simulink model "PIControllerModel"  (R2024b)
settings: Solver=VariableStepAuto  StartTime=0.0  StopTime=10  RelTol=1e-3
values from neighbouring files (symbols this model uses):
  c = 160e-6    (= 0.00016)    [ParamTestSimulationDroop.m]    (also in ParamTestSimulatitestFirstandPI.m)
  Kp_currentLoop = X*r    (= 0.5)    [ParamTestSimulationDroop.m]    (also in ParamTestSimulatitestFirstandPI.m)
  Kp_voltageLoop = Xvoltage/Rc    (= 0.005)    [ParamTestSimulationDroop.m]    (also in ParamTestSimulatitestFirstandPI.m)
  l = 300e-6    (= 0.0003)    [ParamTestSimulationDroop.m]    (also in ParamTestSimulatitestFirstandPI.m)
  r = 0.1    [ParamTestSimulationDroop.m]    (also in ParamTestSimulatitestFirstandPI.m)
  Rc = 1e3    (= 1000)    [ParamTestSimulationDroop.m]    (also in ParamTestSimulatitestFirstandPI.m)
  T32 = sqrt(2/3)*[1 0;-1/2 sqrt(3)/2;-1/2 -sqrt(3)/2]    [ParamTestSimulationDroop.m]    (also in ParamTestSimulatitestFirstandPI.m)
  towI_currentLoop = tow_currnet    (= 0.003)    [ParamTestSimulationDroop.m]    (also in ParamTestSimulatitestFirstandPI.m)
  towI_voltageLoop = tow_voltage    (= 0.16)    [ParamTestSimulationDroop.m]    (also in ParamTestSimulatitestFirstandPI.m)
libraries: spsThreePhaseSeriesRLCBranchLib x7, spsControlledVoltageSourceLib x3, spsThreePhaseVIMeasurementLib x2, spsGroundLib x1, sps_lib x1
settings Model: Creator=manip  LastModifiedBy=rashi
settings SolverCC: AlgebraicLoopSolver=TrustRegion
settings DebuggingCC: UnconnectedInputMsg=warning  UnconnectedOutputMsg=warning  UnconnectedLineMsg=warning
settings ModelReferenceCC: EnableRefExpFcnMdlSchedulingChecks=on
settings RTWCC: GPUComputeCapability=3.5

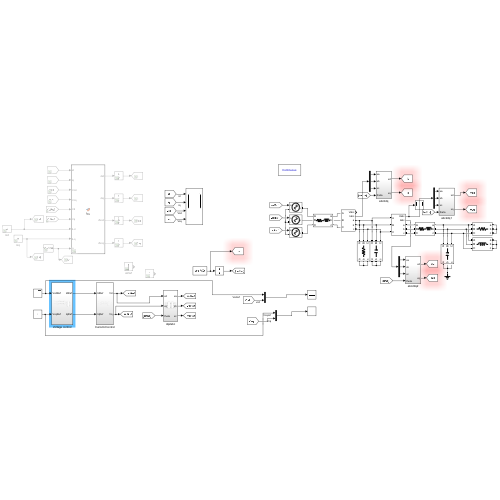
[thumbnail: Simulink's stored preview of the top-level diagram]
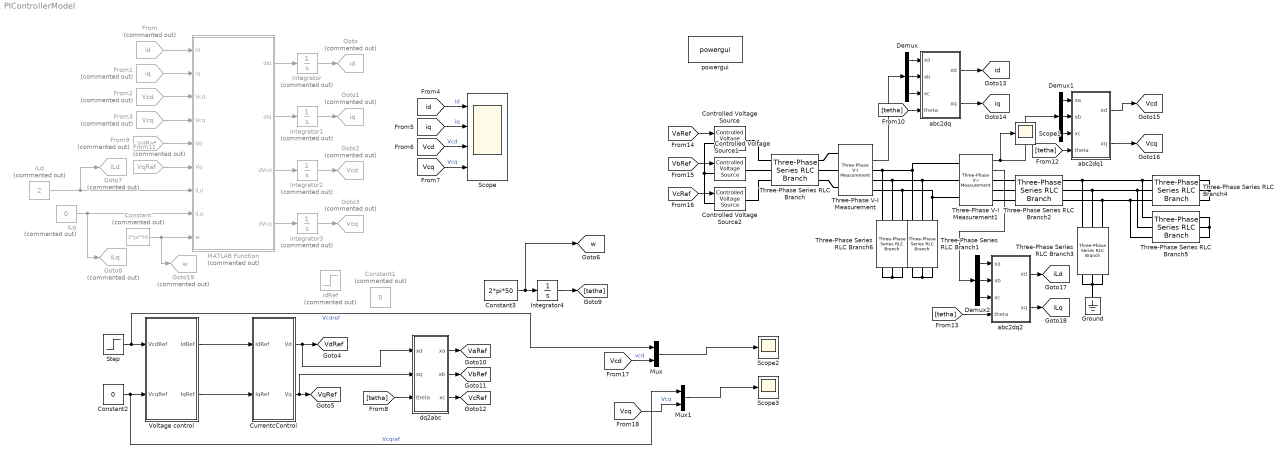
== system PIControllerModel ==
  Constant : Constant  Commented=on  Value=2*pi*50
  Constant1 : Constant  Commented=on  Value=0
  Constant2 : Constant  Value=0
  Constant3 : Constant  Value=2*pi*50
  Controlled Voltage Source : spsControlledVoltageSourceLib/Controlled Voltage Source  Initialize=on  Source_Type=AC  Amplitude=0  Phase=0  Frequency=0  Measurements=None
  Controlled Voltage Source1 : spsControlledVoltageSourceLib/Controlled Voltage Source  Initialize=on  Source_Type=AC  Amplitude=0  Phase=0  Frequency=0  Measurements=None
  Controlled Voltage Source2 : spsControlledVoltageSourceLib/Controlled Voltage Source  Initialize=on  Source_Type=AC  Amplitude=0  Phase=0  Frequency=0  Measurements=None
  CurrentcControl : Subsystem
  Demux : Demux  Outputs=3
  Demux1 : Demux  Outputs=3
  Demux2 : Demux  Outputs=3
  From : From  Commented=on  GotoTag=id  TagVisibility=global
  From1 : From  Commented=on  GotoTag=iq  TagVisibility=global
  From11 : From  Commented=on  GotoTag=VqRef  TagVisibility=global
  From2 : From  Commented=on  GotoTag=Vcd  TagVisibility=global
  From3 : From  Commented=on  GotoTag=Vcq  TagVisibility=global
  From9 : From  Commented=on  GotoTag=VdRef  TagVisibility=global
  Goto : Goto  Commented=on  GotoTag=id  TagVisibility=global
  Goto1 : Goto  Commented=on  GotoTag=iq  TagVisibility=global
  Goto19 : Goto  Commented=on  GotoTag=w  TagVisibility=global
  Goto2 : Goto  Commented=on  GotoTag=Vcd  TagVisibility=global
  Goto3 : Goto  Commented=on  GotoTag=Vcq  TagVisibility=global
  Goto7 : Goto  Commented=on  GotoTag=iLd  TagVisibility=global
  Goto8 : Goto  Commented=on  GotoTag=iLq  TagVisibility=global
  Ground : spsGroundLib/Ground  LConnTagsString=a
  Integrator{,1..3} (4 alike) : Integrator  Commented=on
  Integrator4 : Integrator
  MATLAB Function : MATLAB Function  Commented=on  TreatAsAtomicUnit=on
  Mux : Mux  Inputs=2
  Mux1 : Mux  Inputs=2
  Scope : Scope  NumInputPorts=4
  Scope1 : Scope
  Scope2 : Scope
  Scope3 : Scope
  Step : Step  Time=3  Before=50  After=110  SampleTime=0
  Three-Phase Series RLC Branch : spsThreePhaseSeriesRLCBranchLib/Three-Phase Series RLC Branch  LConnTagsString=A|B|C  RConnTagsString=A|B|C  BranchType=RL  Resistance=r  Inductance=l  Capacitance=1e-6  Measurements=None
  Three-Phase Series RLC Branch1 : spsThreePhaseSeriesRLCBranchLib/Three-Phase Series RLC Branch  LConnTagsString=A|B|C  RConnTagsString=A|B|C  BranchType=C  Resistance=r  Inductance=l  Capacitance=c  Measurements=None
  Three-Phase Series RLC Branch2 : spsThreePhaseSeriesRLCBranchLib/Three-Phase Series RLC Branch  LConnTagsString=A|B|C  RConnTagsString=A|B|C  BranchType=RL  Resistance=1  Inductance=4e-3  Capacitance=1e-6  Measurements=None
  Three-Phase Series RLC Branch3 : spsThreePhaseSeriesRLCBranchLib/Three-Phase Series RLC Branch  LConnTagsString=A|B|C  RConnTagsString=A|B|C  BranchType=C  Resistance=r  Inductance=l  Capacitance=1e-6  Measurements=None
  Three-Phase Series RLC Branch4 : spsThreePhaseSeriesRLCBranchLib/Three-Phase Series RLC Branch  LConnTagsString=A|B|C  RConnTagsString=A|B|C  BranchType=R  Resistance=50  Inductance=4e-3  Capacitance=1e-6  Measurements=None
  Three-Phase Series RLC Branch5 : spsThreePhaseSeriesRLCBranchLib/Three-Phase Series RLC Branch  LConnTagsString=A|B|C  RConnTagsString=A|B|C  BranchType=L  Resistance=50  Inductance=4e-3  Capacitance=1e-6  Measurements=None
  Three-Phase Series RLC Branch6 : spsThreePhaseSeriesRLCBranchLib/Three-Phase Series RLC Branch  LConnTagsString=A|B|C  RConnTagsString=A|B|C  BranchType=R  Resistance=Rc  Inductance=l  Capacitance=c  Measurements=None
  Three-Phase V-I Measurement : spsThreePhaseVIMeasurementLib/Three-Phase V-I Measurement  VoltageMeasurement=phase-to-ground  SetLabelV=off  LabelV=Vabc  Vpu=off  VpuLL=off  CurrentMeasurement=yes  SetLabelI=off  LabelI=Iabc  Ipu=off  Pbase=100e6  Vbase=500e3  OutputType=Complex  PhasorSimulation=off  PSBequivalent=0
  Three-Phase V-I Measurement1 : spsThreePhaseVIMeasurementLib/Three-Phase V-I Measurement  VoltageMeasurement=phase-to-ground  SetLabelV=off  LabelV=Vabc  Vpu=off  VpuLL=off  CurrentMeasurement=yes  SetLabelI=off  LabelI=Iabc  Ipu=off  Pbase=100e6  Vbase=500e3  OutputType=Complex  PhasorSimulation=off  PSBequivalent=0
  Voltage control : Subsystem
  abc2dq : Subsystem
  abc2dq1 : Subsystem
  abc2dq2 : Subsystem
  dq2abc : Subsystem
  iLd : Constant  Commented=on  Value=2
  iLq : Constant  Commented=on  Value=0
  idRef : Step  Commented=on  Time=0.5  Before=2  After=3  SampleTime=0
  powergui : sps_lib/powergui  Priority=1  SimulationMode=Continuous  SampleTime=50e-6  frequency=60  Iterations=50  frequencyindice=0  Pbase=100e6  ErrMax=1e-4  UnitsV=kV  UnitsW=MW  buscounter=0  FunctionMessages=off  echomessages=off  EnableUseOfTLC=off  CurrentSourceSwitches=off  DisableSnubberDevices=off  DisableRonSwitches=off  DisableVfSwitches=off  DisplayEquations=off  AutomaticDiscreteSolvers=off  SolverType=Tustin/Backward Euler (TBE)  Interpol=off  ExternalGateDelay=off  methode=off  Ts=100  x0status=blocks  SPID=on  SwTol=0  HookPort=off  NonlinearTolerance=1e-4  nMaxIteration=100  ContinueOnMaxIteration=off  RestoreLinks=warning  ResistiveCurrentMeasurement=off  Frange=[0:2:500]  Ylog=off  Xlog=on  ShowGrid=off  save=off  variable=ZData  structure=0  ZoomFFT=off  StartTime=0.0  cycles=1  DisplayStyle=1  fundamental=60  FreqAxis=off  MaxFrequency=1000  frequencyindicesteady=1  RmsSteady=1  display=off
  tag scope: VaRef=global, VbRef=global, VcRef=global, Vcd=global, Vcq=global, VdRef=global, VqRef=global, iLd=global, iLq=global, id=global, iq=global, w=global
  wires:
  MATLAB Function/1(did) -> Integrator/1
  MATLAB Function/2(diq) -> Integrator1/1
  MATLAB Function/3(dVcd) -> Integrator2/1
  MATLAB Function/4(dVcq) -> Integrator3/1
  Integrator/1 -> Goto/1
  Integrator1/1 -> Goto1/1
  Integrator2/1 -> Goto2/1
  Integrator3/1 -> Goto3/1
  From/1 -> MATLAB Function/1(id)
  From1/1 -> MATLAB Function/2(iq)
  From3/1 -> MATLAB Function/4(Vcq)
  From2/1 -> MATLAB Function/3(Vcd)
  iLd/1 -> Goto7/1, MATLAB Function/7(iLd)
  iLq/1 -> Goto8/1, MATLAB Function/8(iLq)
  Constant/1 -> Goto19/1, MATLAB Function/9(w)
  [Vcq] -> Scope/4  "Vcq"
  [id] -> Scope/1  "id"
  [iq] -> Scope/2  "iq"
  [Vcd] -> Scope/3  "Vcd"
  From9/1 -> MATLAB Function/5(Vd)
  From11/1 -> MATLAB Function/6(Vq)
  Voltage control/1(IdRef) -> CurrentcControl/1(IdRef)
  Voltage control/2(IqRef) -> CurrentcControl/2(IqRef)
  CurrentcControl/1(Vd) -> dq2abc/1(xd), [VdRef]
  CurrentcControl/2(Vq) -> dq2abc/2(xq), [VqRef]
  Constant2/1 -> Mux1/1, Voltage control/2(VcqRef)  "Vcqref"
  Step/1 -> Mux/1, Voltage control/1(VcdRef)  "Vcdref"
  Constant3/1 -> [w], Integrator4/1
  Integrator4/1 -> [tetha]
  [tetha] -> dq2abc/3(theta)
  dq2abc/1(xa) -> [VaRef]
  dq2abc/2(xb) -> [VbRef]
  dq2abc/3(xc) -> [VcRef]
  Demux/1 -> abc2dq/1(xa)
  Demux/2 -> abc2dq/2(xb)
  Demux/3 -> abc2dq/3(xc)
  Three-Phase V-I Measurement/2 -> Demux/1
  abc2dq/1(xd) -> [id]
  abc2dq/2(xq) -> [iq]
  Three-Phase V-I Measurement1/1 -> Scope1/1, Demux1/1
  Demux1/3 -> abc2dq1/3(xc)
  Demux1/2 -> abc2dq1/2(xb)
  Demux1/1 -> abc2dq1/1(xa)
  abc2dq1/1(xd) -> [Vcd]
  abc2dq1/2(xq) -> [Vcq]
  abc2dq2/2(xq) -> [iLq]
  abc2dq2/1(xd) -> [iLd]
  Three-Phase V-I Measurement1/2 -> Demux2/1
  Demux2/2 -> abc2dq2/2(xb)
  Demux2/3 -> abc2dq2/3(xc)
  Demux2/1 -> abc2dq2/1(xa)
  [tetha] -> abc2dq/4(theta)
  [tetha] -> abc2dq1/4(theta)
  [tetha] -> abc2dq2/4(theta)
  [VaRef] -> Controlled Voltage Source/1
  [VbRef] -> Controlled Voltage Source1/1
  [VcRef] -> Controlled Voltage Source2/1
  [Vcd] -> Mux/2  "vcd"
  Mux1/1 -> Scope3/1
  Mux/1 -> Scope2/1
  [Vcq] -> Mux1/2  "Vcq"
  connections:
  Controlled Voltage Source1/LConn1 -- Controlled Voltage Source/LConn1 -- Controlled Voltage Source2/LConn1
  Three-Phase Series RLC Branch/LConn1 -- Controlled Voltage Source/RConn1
  Three-Phase Series RLC Branch/LConn2 -- Controlled Voltage Source1/RConn1
  Three-Phase Series RLC Branch/LConn3 -- Controlled Voltage Source2/RConn1
  Three-Phase V-I Measurement/LConn1 -- Three-Phase Series RLC Branch/RConn1
  Three-Phase V-I Measurement/LConn2 -- Three-Phase Series RLC Branch/RConn2
  Three-Phase Series RLC Branch/RConn3 -- Three-Phase V-I Measurement/LConn3
  Three-Phase Series RLC Branch1/RConn3 -- Three-Phase Series RLC Branch1/RConn2 -- Three-Phase Series RLC Branch1/RConn1
  Three-Phase Series RLC Branch1/LConn1 -- Three-Phase V-I Measurement1/LConn1 -- Three-Phase Series RLC Branch6/LConn1 -- Three-Phase V-I Measurement/RConn1
  Three-Phase V-I Measurement/RConn2 -- Three-Phase Series RLC Branch6/LConn2 -- Three-Phase V-I Measurement1/LConn2 -- Three-Phase Series RLC Branch1/LConn2
  Three-Phase V-I Measurement/RConn3 -- Three-Phase Series RLC Branch6/LConn3 -- Three-Phase V-I Measurement1/LConn3 -- Three-Phase Series RLC Branch1/LConn3
  Three-Phase V-I Measurement1/RConn1 -- Three-Phase Series RLC Branch2/LConn1
  Three-Phase V-I Measurement1/RConn2 -- Three-Phase Series RLC Branch2/LConn2
  Three-Phase V-I Measurement1/RConn3 -- Three-Phase Series RLC Branch2/LConn3
  Three-Phase Series RLC Branch3/RConn2 -- Three-Phase Series RLC Branch3/RConn3 -- Ground/LConn1 -- Three-Phase Series RLC Branch3/RConn1
  Three-Phase Series RLC Branch2/RConn1 -- Three-Phase Series RLC Branch3/LConn1 -- Three-Phase Series RLC Branch5/LConn1 -- Three-Phase Series RLC Branch4/LConn1
  Three-Phase Series RLC Branch3/LConn2 -- Three-Phase Series RLC Branch2/RConn2 -- Three-Phase Series RLC Branch5/LConn2 -- Three-Phase Series RLC Branch4/LConn2
  Three-Phase Series RLC Branch3/LConn3 -- Three-Phase Series RLC Branch5/LConn3 -- Three-Phase Series RLC Branch4/LConn3 -- Three-Phase Series RLC Branch2/RConn3
  Three-Phase Series RLC Branch4/RConn1 -- Three-Phase Series RLC Branch4/RConn2 -- Three-Phase Series RLC Branch4/RConn3
  Three-Phase Series RLC Branch5/RConn1 -- Three-Phase Series RLC Branch5/RConn2 -- Three-Phase Series RLC Branch5/RConn3
  Three-Phase Series RLC Branch6/RConn3 -- Three-Phase Series RLC Branch6/RConn2 -- Three-Phase Series RLC Branch6/RConn1

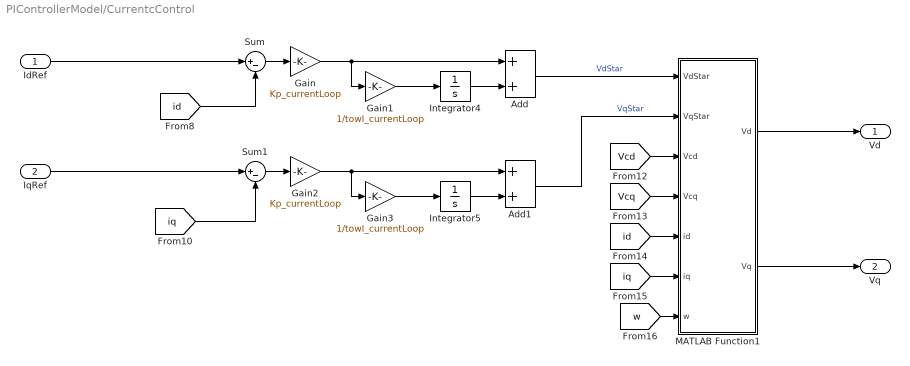
== system PIControllerModel/CurrentcControl ==
  IdRef : Inport
  IqRef : Inport  Port=2
  Add : Sum
  Add1 : Sum
  Gain : Gain  Gain=Kp_currentLoop
  Gain1 : Gain  Gain=1/towI_currentLoop
  Gain2 : Gain  Gain=Kp_currentLoop
  Gain3 : Gain  Gain=1/towI_currentLoop
  Integrator4 : Integrator
  Integrator5 : Integrator
  MATLAB Function1 : MATLAB Function  TreatAsAtomicUnit=on
  Sum : Sum  Inputs=|+-
  Sum1 : Sum  Inputs=|+-
  Vd : Outport
  Vq : Outport  Port=2
  wires:
  [w] -> MATLAB Function1/7(w)
  [iq] -> Sum1/2
  Add/1 -> MATLAB Function1/1(VdStar)  "VdStar"
  [Vcq] -> MATLAB Function1/4(Vcq)
  Gain2/1 -> Gain3/1, Add1/1
  IdRef/1 -> Sum/1
  [id] -> MATLAB Function1/5(id)
  Sum1/1 -> Gain2/1
  Gain3/1 -> Integrator5/1
  Sum/1 -> Gain/1
  IqRef/1 -> Sum1/1
  Add1/1 -> MATLAB Function1/2(VqStar)  "VqStar"
  Integrator5/1 -> Add1/2
  MATLAB Function1/2(Vq) -> Vq/1
  Gain/1 -> Gain1/1, Add/1
  Integrator4/1 -> Add/2
  [Vcd] -> MATLAB Function1/3(Vcd)
  Gain1/1 -> Integrator4/1
  [id] -> Sum/2
  [iq] -> MATLAB Function1/6(iq)
  MATLAB Function1/1(Vd) -> Vd/1

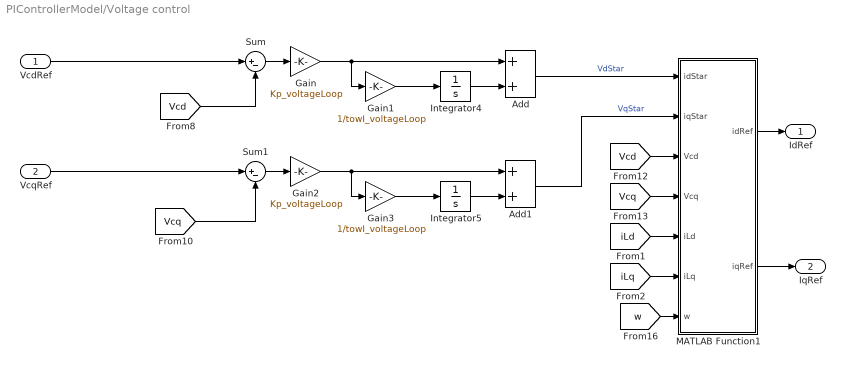
== system PIControllerModel/Voltage control ==
  VcdRef : Inport
  VcqRef : Inport  Port=2
  Add : Sum
  Add1 : Sum
  Gain : Gain  Gain=Kp_voltageLoop
  Gain1 : Gain  Gain=1/towI_voltageLoop
  Gain2 : Gain  Gain=Kp_voltageLoop
  Gain3 : Gain  Gain=1/towI_voltageLoop
  Integrator4 : Integrator
  Integrator5 : Integrator
  MATLAB Function1 : MATLAB Function  TreatAsAtomicUnit=on
  Sum : Sum  Inputs=|+-
  Sum1 : Sum  Inputs=|+-
  IdRef : Outport
  IqRef : Outport  Port=2
  wires:
  Gain/1 -> Gain1/1, Add/1
  Integrator5/1 -> Add1/2
  VcqRef/1 -> Sum1/1
  Sum/1 -> Gain/1
  Gain3/1 -> Integrator5/1
  [iLd] -> MATLAB Function1/5(iLd)
  Sum1/1 -> Gain2/1
  VcdRef/1 -> Sum/1
  [Vcq] -> MATLAB Function1/4(Vcq)
  Gain2/1 -> Gain3/1, Add1/1
  [Vcd] -> Sum/2
  [iLq] -> MATLAB Function1/6(iLq)
  [w] -> MATLAB Function1/7(w)
  Gain1/1 -> Integrator4/1
  [Vcq] -> Sum1/2
  Add1/1 -> MATLAB Function1/2(iqStar)  "VqStar"
  [Vcd] -> MATLAB Function1/3(Vcd)
  Add/1 -> MATLAB Function1/1(idStar)  "VdStar"
  Integrator4/1 -> Add/2
  MATLAB Function1/2(iqRef) -> IqRef/1
  MATLAB Function1/1(idRef) -> IdRef/1

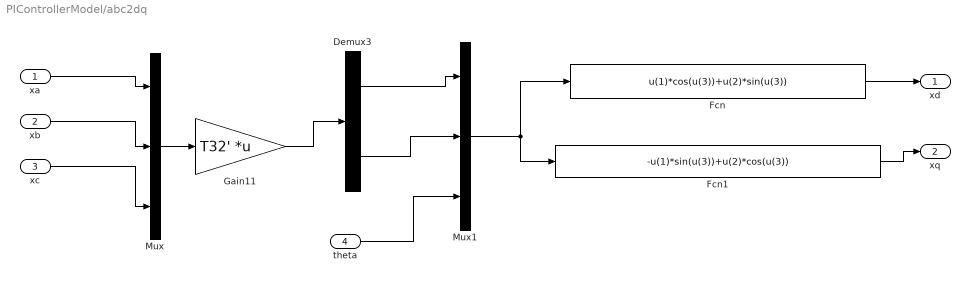
== system PIControllerModel/abc2dq ==
  xa : Inport
  xb : Inport  Port=2
  xc : Inport  Port=3
  theta : Inport  Port=4
  Demux3 : Demux  Outputs=2
  Fcn : Fcn  Expr=u(1)*cos(u(3))+u(2)*sin(u(3))
  Fcn1 : Fcn  Expr=-u(1)*sin(u(3))+u(2)*cos(u(3))
  Gain11 : Gain  Gain=T32'  Multiplication=Matrix(K*u)
  Mux : Mux  Inputs=3
  Mux1 : Mux  Inputs=3
  xd : Outport
  xq : Outport  Port=2
  wires:
  Fcn1/1 -> xq/1
  theta/1 -> Mux1/3
  xb/1 -> Mux/2
  Mux/1 -> Gain11/1
  Gain11/1 -> Demux3/1
  xc/1 -> Mux/3
  Mux1/1 -> Fcn/1, Fcn1/1
  Fcn/1 -> xd/1
  xa/1 -> Mux/1
  Demux3/1 -> Mux1/1
  Demux3/2 -> Mux1/2

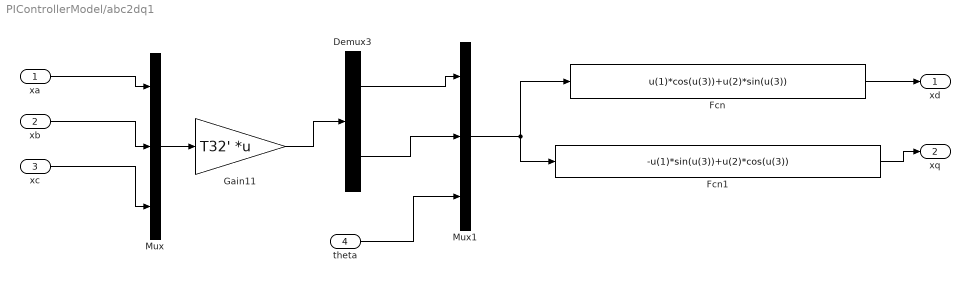
== system PIControllerModel/abc2dq1 ==
  xa : Inport
  xb : Inport  Port=2
  xc : Inport  Port=3
  theta : Inport  Port=4
  Demux3 : Demux  Outputs=2
  Fcn : Fcn  Expr=u(1)*cos(u(3))+u(2)*sin(u(3))
  Fcn1 : Fcn  Expr=-u(1)*sin(u(3))+u(2)*cos(u(3))
  Gain11 : Gain  Gain=T32'  Multiplication=Matrix(K*u)
  Mux : Mux  Inputs=3
  Mux1 : Mux  Inputs=3
  xd : Outport
  xq : Outport  Port=2
  wires:
  Demux3/2 -> Mux1/2
  Demux3/1 -> Mux1/1
  xa/1 -> Mux/1
  Fcn/1 -> xd/1
  Mux1/1 -> Fcn1/1, Fcn/1
  xc/1 -> Mux/3
  Gain11/1 -> Demux3/1
  Mux/1 -> Gain11/1
  xb/1 -> Mux/2
  theta/1 -> Mux1/3
  Fcn1/1 -> xq/1

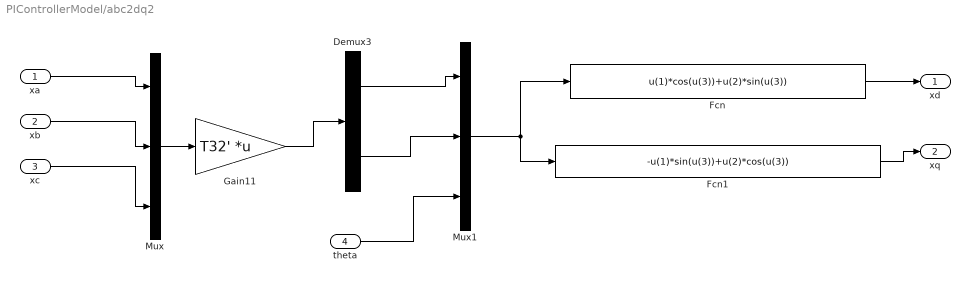
== system PIControllerModel/abc2dq2 ==
  xa : Inport
  xb : Inport  Port=2
  xc : Inport  Port=3
  theta : Inport  Port=4
  Demux3 : Demux  Outputs=2
  Fcn : Fcn  Expr=u(1)*cos(u(3))+u(2)*sin(u(3))
  Fcn1 : Fcn  Expr=-u(1)*sin(u(3))+u(2)*cos(u(3))
  Gain11 : Gain  Gain=T32'  Multiplication=Matrix(K*u)
  Mux : Mux  Inputs=3
  Mux1 : Mux  Inputs=3
  xd : Outport
  xq : Outport  Port=2
  wires:
  Fcn1/1 -> xq/1
  theta/1 -> Mux1/3
  xb/1 -> Mux/2
  Mux/1 -> Gain11/1
  Gain11/1 -> Demux3/1
  xc/1 -> Mux/3
  Mux1/1 -> Fcn/1, Fcn1/1
  Fcn/1 -> xd/1
  xa/1 -> Mux/1
  Demux3/1 -> Mux1/1
  Demux3/2 -> Mux1/2

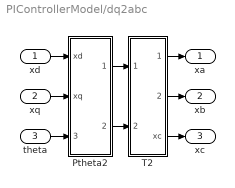
== system PIControllerModel/dq2abc ==
  xd : Inport
  xq : Inport  Port=2
  theta : Inport  Port=3
  Ptheta2 : Subsystem
  T2 : Subsystem
  xa : Outport
  xb : Outport  Port=2
  xc : Outport  Port=3
  wires:
  xq/1 -> Ptheta2/2(xq)
  Ptheta2/2(xbeta) -> T2/2(xbeta)
  T2/1(xa) -> xa/1
  T2/3(xc) -> xc/1
  Ptheta2/1(xalpha) -> T2/1(xalpha)
  xd/1 -> Ptheta2/1(xd)
  theta/1 -> Ptheta2/3(theta)
  T2/2(xb) -> xb/1

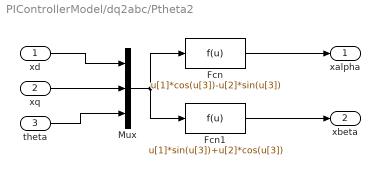
== system PIControllerModel/dq2abc/Ptheta2 ==
  xd : Inport
  xq : Inport  Port=2
  theta : Inport  Port=3
  Fcn : Fcn  Expr=u[1]*cos(u[3])-u[2]*sin(u[3])
  Fcn1 : Fcn  Expr=u[1]*sin(u[3])+u[2]*cos(u[3])
  Mux : Mux  Inputs=3
  xalpha : Outport
  xbeta : Outport  Port=2
  wires:
  xq/1 -> Mux/2
  xd/1 -> Mux/1
  Mux/1 -> Fcn1/1, Fcn/1
  Fcn1/1 -> xbeta/1
  Fcn/1 -> xalpha/1
  theta/1 -> Mux/3

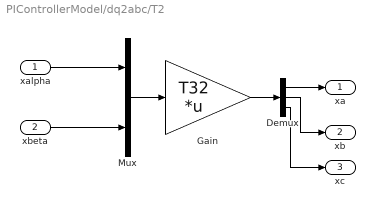
== system PIControllerModel/dq2abc/T2 ==
  xalpha : Inport
  xbeta : Inport  Port=2
  Demux : Demux  Outputs=3
  Gain : Gain  Gain=T32  Multiplication=Matrix(K*u)
  Mux : Mux  Inputs=2
  xa : Outport
  xb : Outport  Port=2
  xc : Outport  Port=3
  wires:
  Demux/3 -> xc/1
  Demux/2 -> xb/1
  Demux/1 -> xa/1
  Gain/1 -> Demux/1
  Mux/1 -> Gain/1
  xalpha/1 -> Mux/1
  xbeta/1 -> Mux/2

== matlab function PIControllerModel/CurrentcControl/MATLAB Function1 ==
  data: VdStar input; Vd output; VqStar input; Vcd input; Vcq input; id input; iq input; w input; Vq output; l parameter
function [Vd,Vq] = fcn(VdStar,VqStar,Vcd,Vcq,id,iq,w, l)

Vd = VdStar-l*w*iq+Vcd;
Vq = VqStar+l*w*id+Vcq;

== matlab function PIControllerModel/MATLAB Function ==
  data: id input; did output; iq input; Vcd input; Vcq input; Vd input; Vq input; iLd input; iLq input; w input; diq output; dVcd output; dVcq output; r parameter; l parameter; c parameter; Rc parameter
function [did,diq,dVcd,dVcq] = fcn(id,iq,Vcd,Vcq,Vd,Vq,iLd,iLq,w,r, l, c, Rc)
did = (Vd-Vcd-r*id+l*w*iq)/l;
diq = (Vq-Vcq-r*iq-l*w*id)/l;
dVcd = (id-iLd+c*w*Vcq-Vcd/Rc)/c;
dVcq = (iq-iLq-c*w*Vcd-Vcq/Rc)/c;

== matlab function PIControllerModel/Voltage control/MATLAB Function1 ==
  data: idStar input; idRef output; iqStar input; Vcd input; Vcq input; iLd input; iLq input; w input; iqRef output; c parameter
function [idRef,iqRef] = fcn(idStar,iqStar,Vcd,Vcq,iLd,iLq,w, c)


idRef = idStar+iLd-c*w*Vcq;
iqRef = iqStar+iLq+c*w*Vcd;
